simulink model "proj2exampleMinh"  (R2017b)
settings: Solver=VariableStepAuto  StartTime=0.0  StopTime=inf  RelTol=1e-3
libraries: libraryProject2 x3, LibraryBlock x1, realtime_pacer_lib x1
settings Model: Creator=BRAHIMA FANNY  LastModifiedBy=minh
settings CodeAppCC: StateflowObjectComments=on

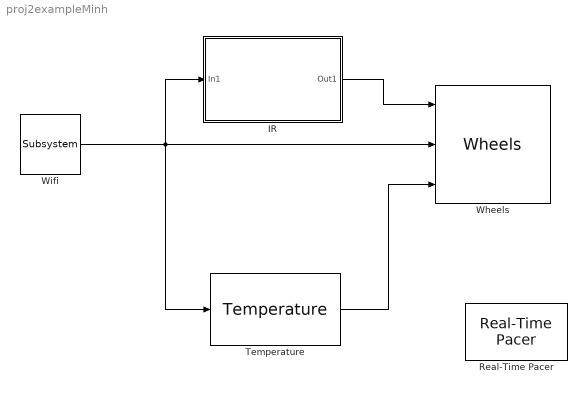
== system proj2exampleMinh ==
  "IR " : Subsystem  AncestorBlock=libraryProject2/IR
  Real-Time Pacer : realtime_pacer_lib/Real-Time Pacer  simTimePerRealTime=.5
  Temperature : libraryProject2/Temperature
  Wheels : libraryProject2/Wheels
  Wifi : libraryProject2/Subsystem
  wires:
  "IR "/1(Out1) -> Wheels/1
  Temperature/1 -> Wheels/3
  Wifi/1 -> Temperature/1, Wheels/2, "IR "/1(In1)

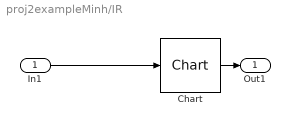
== system proj2exampleMinh/IR  ==
  In1 : Inport
  Chart : LibraryBlock/ir /Chart
  Out1 : Outport
  wires:
  In1/1 -> Chart/1
  Chart/1 -> Out1/1
